simulink model "paper_aims"  (R2022a)
settings: Solver=ode23  StartTime=0.00  StopTime=T  MaxStep=0.1  RelTol=1e-3
values from neighbouring files (symbols this model uses):
  a = (v([2:end 1],:)-v([end 1:end-1],:))./T./2    [elvio_resample.m]
  k = kp.*0    [stat_k.m]
  k_av = [1;2*v0;v0^2]*kp_av    [stat_k.m]
  v = interp1(ct,cv,t)    [elvio_resample.m]
undefined symbols (not defined in the file or in its folder): alpha, c, m, x
settings Model: Creator=thomas  LastModifiedBy=thomas

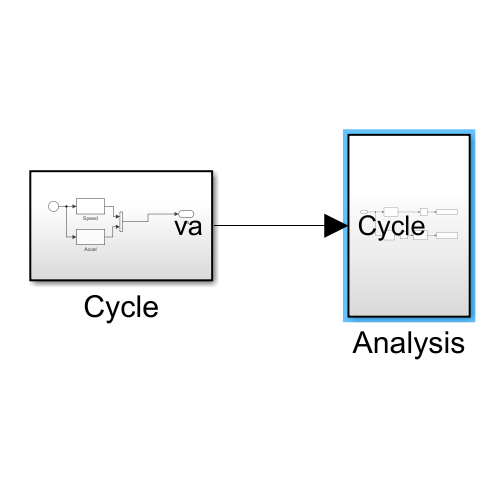
[thumbnail: Simulink's stored preview of the top-level diagram]
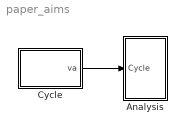
== system paper_aims ==
  Analysis : Subsystem
  Cycle : Subsystem
  wires:
  Cycle/1(va) -> Analysis/1(Cycle)

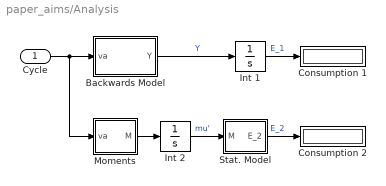
== system paper_aims/Analysis ==
  Cycle : Inport
  Backwards Model : Subsystem
  Consumption 1 : Display
  Consumption 2 : Display
  Int 1 : Integrator
  Int 2 : Integrator
  Moments : Subsystem
  Stat. Model : Subsystem
  wires:
  Cycle/1 -> Moments/1(va), Backwards Model/1(va)
  Int 1/1 -> Consumption 1/1  "E_1"
  Int 2/1 -> Stat. Model/1(M)  "mu'"
  Moments/1(M) -> Int 2/1
  Stat. Model/1(E_2) -> Consumption 2/1  "E_2"
  Backwards Model/1(Y) -> Int 1/1  "Y"

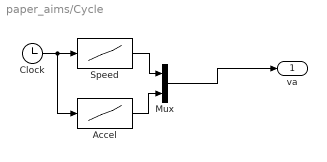
== system paper_aims/Cycle ==
  Accel : Lookup_n-D  NumberOfTableDimensions=1  BreakpointsForDimension1=x  Table=a  InterpMethod=Flat  ExtrapMethod=Clip  InternalRulePriority=Speed  RndMeth=Simplest
  Clock : Clock
  Mux : Mux  Inputs=2
  Speed : Lookup_n-D  NumberOfTableDimensions=1  BreakpointsForDimension1=x  Table=v  ExtrapMethod=Clip  InternalRulePriority=Speed  RndMeth=Simplest
  va : Outport
  wires:
  Accel/1 -> Mux/2
  Clock/1 -> Accel/1, Speed/1
  Speed/1 -> Mux/1
  Mux/1 -> va/1

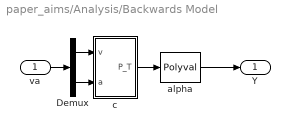
== system paper_aims/Analysis/Backwards Model ==
  va : Inport
  Demux : Demux  Outputs=2
  alpha : Polyval  Coefs=alpha
  c : Subsystem
  Y : Outport
  wires:
  c/1(P_T) -> alpha/1
  Demux/1 -> c/1(v)
  Demux/2 -> c/2(a)
  alpha/1 -> Y/1
  va/1 -> Demux/1

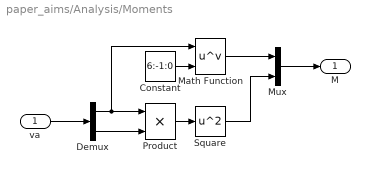
== system paper_aims/Analysis/Moments ==
  va : Inport
  Constant : Constant  Value=6:-1:0
  Demux : Demux  Outputs=2
  Math Function : Math  Operator=pow
  Mux : Mux  Inputs=2
  Product : Product
  Square : Math  Operator=square
  M : Outport
  wires:
  Mux/1 -> M/1
  Constant/1 -> Math Function/2
  Product/1 -> Square/1
  Square/1 -> Mux/2
  Math Function/1 -> Mux/1
  Demux/1 -> Math Function/1, Product/1
  Demux/2 -> Product/2
  va/1 -> Demux/1

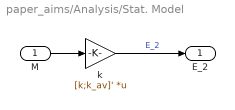
== system paper_aims/Analysis/Stat. Model ==
  M : Inport
  k : Gain  Gain=[k;k_av]'  Multiplication=Matrix(K*u)
  E_2 : Outport
  wires:
  M/1 -> k/1
  k/1 -> E_2/1  "E_2"

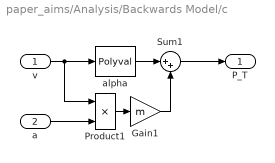
== system paper_aims/Analysis/Backwards Model/c ==
  v : Inport
  a : Inport  Port=2
  Gain1 : Gain  Gain=m
  Product1 : Product
  Sum1 : Sum  Inputs=|++
  alpha : Polyval  Coefs=[c 0]
  P_T : Outport
  wires:
  Product1/1 -> Gain1/1
  Gain1/1 -> Sum1/2
  alpha/1 -> Sum1/1
  v/1 -> Product1/1, alpha/1
  Sum1/1 -> P_T/1
  a/1 -> Product1/2
